simulink model "P1_Ex5"  (R2021a)
settings: Solver=FixedStepAuto  StartTime=0.0  StopTime=Total_time  RelTol=1e-3
PreLoadFcn:
  | PreLoad_P1_Ex5
StopFcn:
  | post_P1_Ex5
undefined symbols (not defined in the file): Kp, Tg, Ts
libraries: arduinolib x4
settings Model: SimulationMode=external  ExtModeTrigDuration=2  Creator=Eneko Lerma  LastModifiedBy=UPCnet
settings SolverCC: AlgebraicLoopSolver=TrustRegion
settings DataIOCC: ReturnWorkspaceOutputs=off
settings OptimizationCC: EnhancedBackFolding=on  PassReuseOutputArgsAs=Individual arguments  MaxStackSize=64  OptimizeBlockOrder=speed  DifferentSizesBufferReuse=on  OptimizationCustomize=off  EfficientTunableParamExpr=on
settings DebuggingCC: ParameterPrecisionLossMsg=none  ParameterTunabilityLossMsg=error  SFMachineParentedDataDiag=warning  ArithmeticOperatorsInVariantConditions=warning
settings HardwareCC: ProdBitPerPointer=32  ProdBitPerSizeT=32  ProdBitPerPtrDiffT=32  ProdLargestAtomicInteger=Long  ProdLargestAtomicFloat=Double  ProdWordSize=32  ProdHWDeviceType=ARM Compatible->ARM Cortex
settings SFSimCC: SimUseLocalCustomCode=off  MATLABDynamicMemAlloc=off  CustomCodeUndefinedFunction=UseInterfaceOnly
settings RTWCC: SystemTargetFile=ert.tlc  HardwareBoard=Arduino Due  TemplateMakefile=ert_default_tmf  GenerateReport=on  RTWUseLocalCustomCode=off  Toolchain=Arduino ARM  BuildConfiguration=Faster Runs  IncludeHyperlinkInReport=on  LaunchReport=on  GenerateTraceInfo=on  GenerateTraceReport=on  GenerateTraceReportSl=on  GenerateTraceReportSf=on  GenerateTraceReportEml=on
settings RTWCC: CustomTerminator=|
  | writeDigitalPin((uint8_T)3, 0);
  | writeDigitalPin((uint8_T)5, 0);
settings CodeAppCC: ForceParamTrailComments=on  IgnoreCustomStorageClasses=off  OperatorAnnotations=on  SimulinkDataObjDesc=on  SFDataObjDesc=on  InsertBlockDesc=on
settings ERTTargetCC: SupportContinuousTime=on  SupportVariableSizeSignals=on

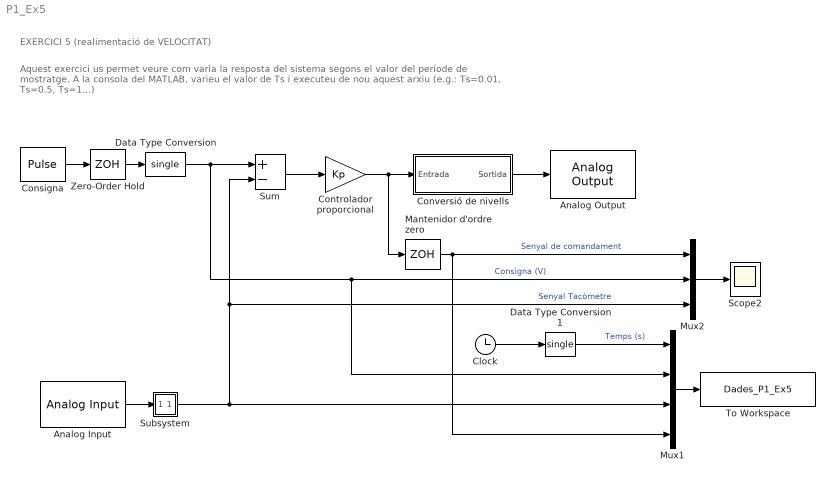
== system P1_Ex5 ==
  note: Aquest exercici us permet veure com varia la resposta del sistema segons el valor del període de mostratge.
      | A la consola del MATLAB, varieu el valor de Ts i executeu de nou aquest arxiu (e.g.: Ts=0.01, Ts=0.5, Ts=1...)
  note: EXERCICI 5 (realimentació de VELOCITAT)
  Analog Input : arduinolib/Analog Input  pinNumber=0  ReadResultsOnly=off  ConversionTriggerSource=Software  ExternalTriggerType=uint32(0)  OutputDataType=uint16  EnableConversionCompleteNotify=off  EnableOuputStatus=off  SampleTime=Tg  blockPlatform=arduino
  Analog Output : arduinolib/Analog Output  DACpin=DAC1  blockPlatform=arduino
      settings: SourceProductBaseCode=ARDUINO
  Clock : Clock
  Consigna : DiscretePulseGenerator  PulseType=Time based  Amplitude=2  Period=8  PulseWidth=50
  Controlador proporcional : Gain  Gain=Kp  OutDataTypeStr=single
  Conversió de nivells : Subsystem
  Data Type Conversion : DataTypeConversion  OutDataTypeStr=single
  Data Type Conversion1 : DataTypeConversion  OutDataTypeStr=single
  Mantenidor d'ordre zero : ZeroOrderHold  SampleTime=Ts
  Mux1 : Mux
  Mux2 : Mux  Inputs=3
  Scope2 : Scope
  Subsystem : Subsystem
  Sum : Sum  Inputs=+-
  To Workspace : ToWorkspace  VariableName=Dades_P1_Ex5  SampleTime=-1
  Zero-Order Hold : ZeroOrderHold  SampleTime=Ts
  wires:
  Conversió de nivells/1(Sortida) -> Analog Output/1
  Sum/1 -> Controlador proporcional/1
  Controlador proporcional/1 -> Conversió de nivells/1(Entrada), Mantenidor d'ordre zero/1
  Zero-Order Hold/1 -> Data Type Conversion/1
  Mux1/1 -> To Workspace/1
  Mux2/1 -> Scope2/1
  Mantenidor d'ordre zero/1 -> Mux2/1, Mux1/4  "Senyal de comandament"
  Clock/1 -> Data Type Conversion1/1
  Data Type Conversion/1 -> Sum/1, Mux1/2, Mux2/2  "Consigna (V)"
  Consigna/1 -> Zero-Order Hold/1
  Data Type Conversion1/1 -> Mux1/1  "Temps (s)"
  Subsystem/1("  ") -> Sum/2, Mux2/3, Mux1/3  "Senyal Tacòmetre"
  Analog Input/1 -> Subsystem/1(" ")

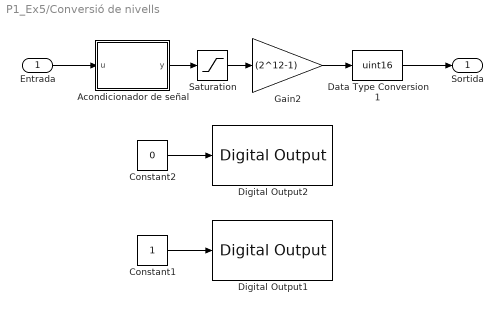
== system P1_Ex5/Conversió de nivells ==
  Entrada : Inport  OutDataTypeStr=single
  Acondicionador de señal : MATLAB Function  TreatAsAtomicUnit=on
  Constant1 : Constant
  Constant2 : Constant  Value=0
  Data Type Conversion1 : DataTypeConversion  OutDataTypeStr=uint16
  Digital Output1 : arduinolib/Digital Output  pinNumber=5  Direction=output  blockPlatform=arduino
  Digital Output2 : arduinolib/Digital Output  pinNumber=3  Direction=output  blockPlatform=arduino
  Gain2 : Gain  Gain=(2^12-1)  OutDataTypeStr=single
  Saturation : Saturate  UpperLimit=1  LowerLimit=0  OutDataTypeStr=single
  Sortida : Outport  OutDataTypeStr=uint16  VectorParamsAs1DForOutWhenUnconnected=off
  wires:
  Saturation/1 -> Gain2/1
  Data Type Conversion1/1 -> Sortida/1
  Acondicionador de señal/1(y) -> Saturation/1
  Entrada/1 -> Acondicionador de señal/1(u)
  Gain2/1 -> Data Type Conversion1/1
  Constant1/1 -> Digital Output1/1
  Constant2/1 -> Digital Output2/1

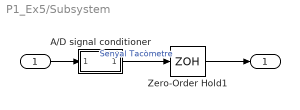
== system P1_Ex5/Subsystem ==
  " " : Inport
  A/D signal conditioner : Subsystem
  Zero-Order Hold1 : ZeroOrderHold  SampleTime=Ts
  "  " : Outport  VectorParamsAs1DForOutWhenUnconnected=off
  wires:
  A/D signal conditioner/1(" ") -> Zero-Order Hold1/1  "Senyal Tacòmetre"
  Zero-Order Hold1/1 -> "  "/1
  " "/1 -> A/D signal conditioner/1(" ")

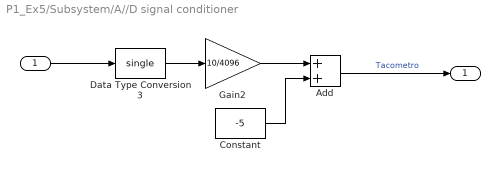
== system P1_Ex5/Subsystem/A//D signal conditioner ==
  " " : Inport
  Add : Sum  AccumDataTypeStr=single
  Constant : Constant  Value=-5  OutDataTypeStr=single
  Data Type Conversion3 : DataTypeConversion  OutDataTypeStr=single
  Gain2 : Gain  Gain=10/4096  OutDataTypeStr=single
  " " : Outport  VectorParamsAs1DForOutWhenUnconnected=off
  wires:
  " "/1 -> Data Type Conversion3/1
  Add/1 -> " "/1  "Tacometro"
  Gain2/1 -> Add/1
  Constant/1 -> Add/2
  Data Type Conversion3/1 -> Gain2/1

== matlab function P1_Ex5/Conversió de nivells/Acondicionador de señal ==
  data: u input; y output
function y = fcn(u)
y =0.0968*u+0.5058;
